simulink model "AM_SSB_LC"  (R2024a)
settings: Solver=VariableStepAuto  StartTime=0.0  StopTime=10.0  RelTol=1e-3
settings Model: Creator=zeyad  LastModifiedBy=zeyad

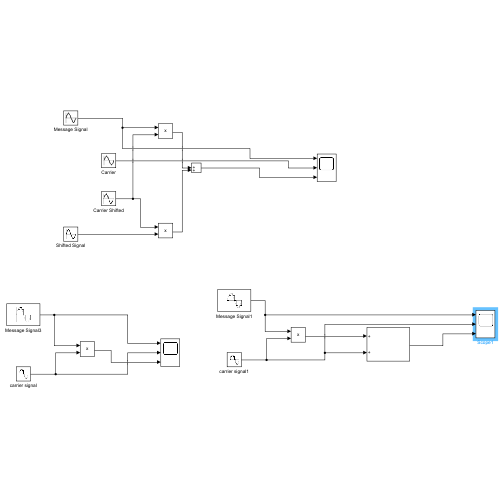
[thumbnail: Simulink's stored preview of the top-level diagram]
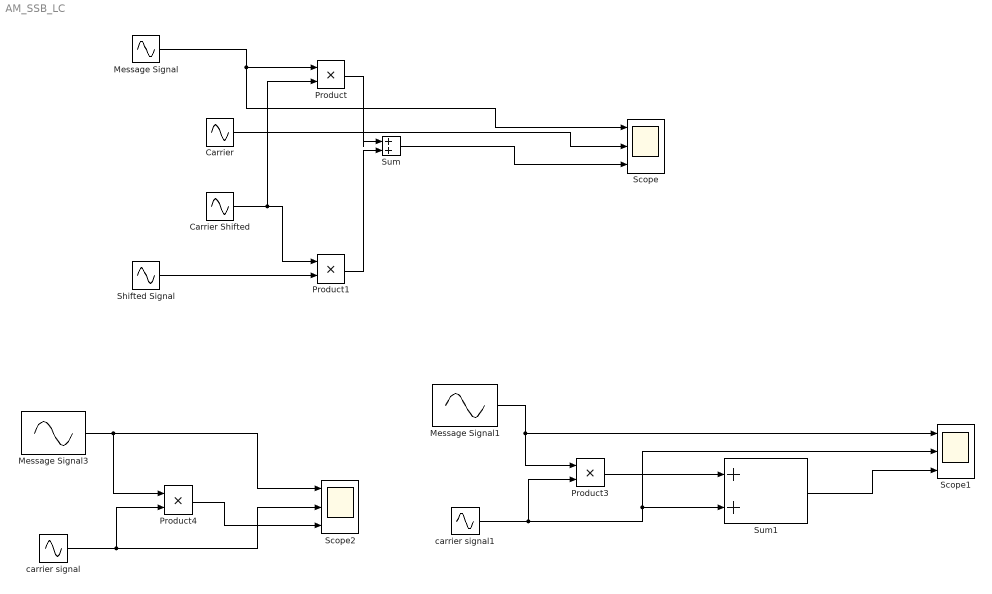
== system AM_SSB_LC ==
  Carrier : Sin  Frequency=100  SampleTime=0
  Carrier Shifted : Sin  Frequency=100  Phase=-(pi/2)  SampleTime=0
  Message Signal : Sin  Frequency=5  SampleTime=0
  Message Signal1 : Sin  Amplitude=2  Frequency=5  SampleTime=1/1000
  Message Signal3 : Sin  Frequency=5  SampleTime=1/1000
  Product{,1,3..4} (4 alike) : Product
  Scope : Scope  NumInputPorts=3
  Scope1 : Scope  NumInputPorts=3
  Scope2 : Scope  NumInputPorts=3
  Shifted Signal : Sin  Frequency=5  Phase=-(pi/2)  SampleTime=0
  Sum : Sum  Inputs=|++
  Sum1 : Sum
  carrier signal : Sin  Frequency=50  SampleTime=1/1000
  carrier signal1 : Sin  Amplitude=3  Frequency=50  SampleTime=1/1000
  wires:
  Product/1 -> Sum/1
  Product1/1 -> Sum/2
  Message Signal/1 -> Scope/1, Product/1
  Shifted Signal/1 -> Product1/2
  Carrier Shifted/1 -> Product/2, Product1/1
  Message Signal1/1 -> Product3/1, Scope1/1
  carrier signal1/1 -> Product3/2, Scope1/2, Sum1/2
  Product3/1 -> Sum1/1
  Sum1/1 -> Scope1/3
  carrier signal/1 -> Product4/2, Scope2/2
  Message Signal3/1 -> Product4/1, Scope2/1
  Product4/1 -> Scope2/3
  Sum/1 -> Scope/3
  Carrier/1 -> Scope/2
